simulink model "twoAWGNChannelEffect"  (R2018a)
settings: Solver=VariableStepAuto  StartTime=0.0  StopTime=0.5  RelTol=1e-3
undefined symbols (not defined in the file): DiscIntNeverNeededParam
libraries: commchan3 x1, dsparch4 x1, commsynccomp2 x1, dspsrcs4 x1
settings Model: Creator=Neo  LastModifiedBy=Neo

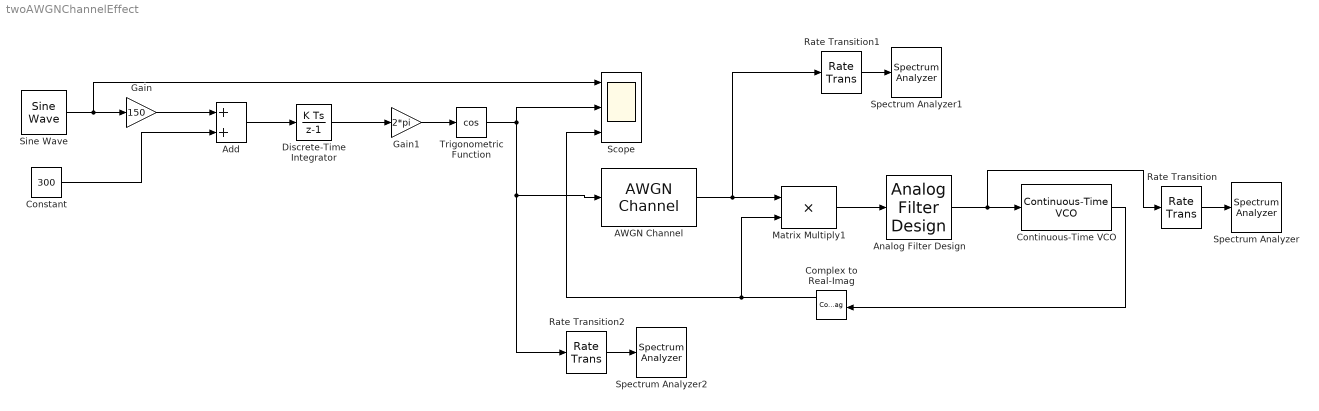
== system twoAWGNChannelEffect ==
  AWGN Channel : commchan3/AWGN Channel  InputProcessing=Columns as channels (frame based)  seed=67  noiseMode=Variance from mask  EbNodB=10  EsNodB=10  SNRdB=10  bitsPerSym=1  Ps=1  Tsym=1  variance=20
  Add : Sum
  Analog Filter Design : dsparch4/Analog Filter Design  method=Butterworth  filttype=Lowpass  N=10  Wlo=2*pi*600  Whi=80  Rp=2  Rs=40
  Complex to Real-Imag : ComplexToRealImag
  Constant : Constant  Value=300
  Continuous-Time VCO : commsynccomp2/Continuous-Time VCO  Ac=1  Fc=10  Kc=50  Ph=0
      settings: SourceProductName=Communications System Toolbox  SourceProductBaseCode=CM
  Discrete-Time Integrator : DiscreteIntegrator  gainval=1  SampleTime=1/98000  ICPrevOutput=DiscIntNeverNeededParam  ICPrevScaledInput=DiscIntNeverNeededParam
  Gain : Gain  Gain=150
  Gain1 : Gain  Gain=2*pi
  Matrix Multiply1 : Product
  Rate Transition : RateTransition  OutPortSampleTime=1/98000
  Rate Transition1 : RateTransition  OutPortSampleTime=1/98000
  Rate Transition2 : RateTransition  OutPortSampleTime=1/98000
  Scope : Scope  NumInputPorts=3
  Sine Wave : dspsrcs4/Sine Wave  Amplitude=1  Frequency=10  Phase=90  SampleMode=Discrete  OutComplex=Real  CompMethod=Trigonometric fcn  TableSize=Speed  SampleTime=1/98000  SamplesPerFrame=1  ResetState=Restart at time zero  OutputFrames=off  dataType=double  wordLen=16  udDataType=sfix(16)  fracBitsMode=Best precision  numFracBits=15  OutDataTypeStr=double  LastOutDataTypeStr=double
  Spectrum Analyzer : SpectrumAnalyzer
  Spectrum Analyzer1 : SpectrumAnalyzer
  Spectrum Analyzer2 : SpectrumAnalyzer
  Trigonometric Function : Trigonometry  Operator=cos
  wires:
  Continuous-Time VCO/1 -> Complex to Real-Imag/1
  Constant/1 -> Add/2
  Matrix Multiply1/1 -> Analog Filter Design/1
  Analog Filter Design/1 -> Rate Transition/1, Continuous-Time VCO/1
  Complex to Real-Imag/1 -> Matrix Multiply1/2, Scope/3
  Sine Wave/1 -> Scope/1, Gain/1
  Add/1 -> Discrete-Time Integrator/1
  Gain1/1 -> Trigonometric Function/1
  Discrete-Time Integrator/1 -> Gain1/1
  Gain/1 -> Add/1
  Rate Transition/1 -> Spectrum Analyzer/1
  Rate Transition1/1 -> Spectrum Analyzer1/1
  Trigonometric Function/1 -> AWGN Channel/1, Rate Transition2/1, Scope/2
  Rate Transition2/1 -> Spectrum Analyzer2/1
  AWGN Channel/1 -> Rate Transition1/1, Matrix Multiply1/1
